simulink model "CompleteDronePathSimulation2"  (R2022b)
settings: Solver=VariableStepAuto  StartTime=0.0  StopTime=10.0  RelTol=1e-3
settings Model: Creator=zs  LastModifiedBy=zs

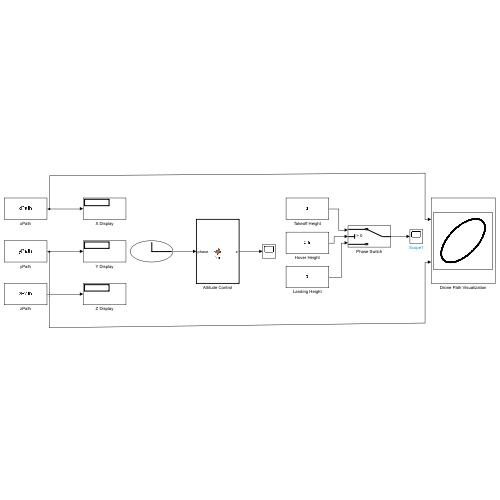
[thumbnail: Simulink's stored preview of the top-level diagram]
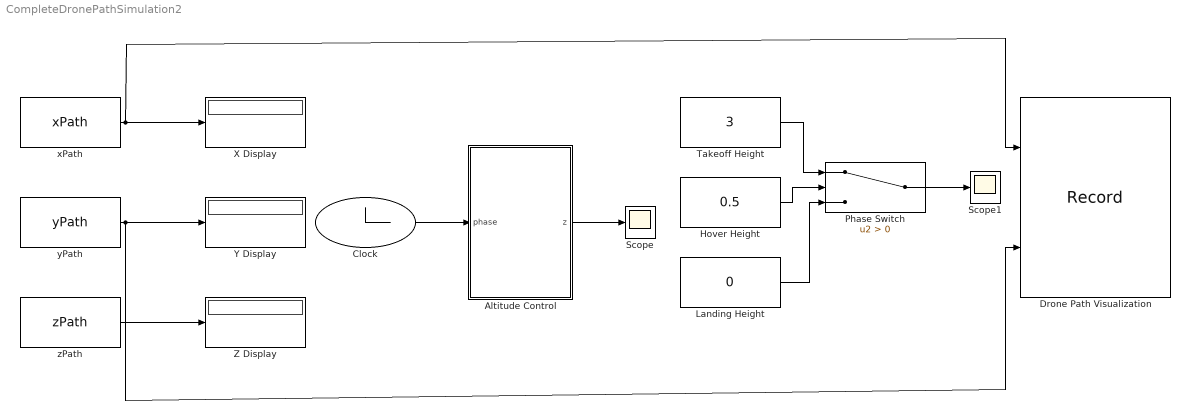
== system CompleteDronePathSimulation2 ==
  Altitude Control : MATLAB Function  TreatAsAtomicUnit=on
  Clock : Clock
  Drone Path Visualization : Record  FileSettingsInternal="{\"entries\":[{\"content\":{\"excelSettings\":{\"content\":{},\"type\":\"Streamout.ExcelSettings\"}},\"type\":\"Streamout.FileSettingStorage\",\"uuid\":\"701c7f2f-fa6d-4916-bfb4-89bd70d8efd9\"}],\"packageUris\":[\"http://schema.mathworks.com/mf0/streamout_blocks/R2020a\"],\"version\":\"1.0\"}"  Layout=[1 1]  SignalsInternal="{\"entries\":[{\"content\":{\"signals\":[{\"content\":{\"blockPath\":[\"CompleteDronePathSimulation2/Drone Path Visualization\"],\"channel\":[],\"dimensions\":[179],\"domain\":\"CompleteDronePathSimulation2/Drone Path Visualization\",\"hasChildren\":true,\"lineColor\":\"#edb120\",\"plots\":[],\"port\":1,\"sid\":[],\"signalID\":225,\"signalName\":\"xPath\"},\"type\":\"RecordBlkView.Signal\",\"uuid\":\"a3cad74d-0c4d-46ad-b448-e85591da0594\"},{\"content\":{\"blockPath\":[\"CompleteDronePathSimulation2/Drone Path Visualization\"],\"channel\":[1],\"dimensions\":[179],\"domain\":\"CompleteDronePathSimulation2/Drone Path Visualization\",\"lineColor\":\"#7e2f8e\",\"parentID\":225,\"plots\":[],\"port\":1,\"sid\":[],\"signalID\":226,\"signalName\":\"xPath\"},\"type\":\"RecordBlkView.Signal\",\"uuid\":\"7178f454-a0ae-4261-bb45-d0e300f4410c\"},{\"content\":{\"blockPath\":[\"CompleteDronePathSimulation2/Drone Path Visualization\"],\"channel\":[],\"dimensions\":[179],\"domain\":\"CompleteDronePathSimulation2/Drone Path Visualization\",\"hasChildren\":true,\"lineColor\":\"#77ac30\",\"plots\":[],\"port\":2,\"sid\":[],\"signalID\":408,\"signalName\":\"yPath\"},\"type\":\"RecordBlkView.Signal\",\"uuid\":\"60e1e068-7377-4912-8406-220e7cc34102\"},{\"content\":{\"blockPath\":[\"CompleteDronePathSimulation2/Drone Path Visualization\"],\"channel\":[1],\"dimensions\":[179],\"domain\":\"CompleteDronePathSimulation2/Drone Path Visualization\",\"lineColor\":\"#4dbeee\",\"parentID\":408,\"plots\":[],\"port\":2,\"sid\":[],\"signalID\":409,\"signalName\":\"yPath\"},\"type\":\"RecordBlkView.Signal\",\"uuid\":\"6962e288-c15f-4001-a316-d17ff70b3f4c\"}]},\"type\":\"RecordBlkView.InputSignals\",\"uuid\":\"a07fd186-7fd0-4c18-bff8-9bf155d2cde3\"}],\"packageUris\":[\"http://schema.mathworks.com/mf0/streamout_blocks/R2020a\"],\"version\":\"1.0\"}"  VisualizationBindings="{\"xyplotplugin\":{\"info\":[{\"series\":[],\"subplotID\":1}]}}"  CompatibilityTag=XY
  Hover Height : Constant  Value=0.5
  Landing Height : Constant  Value=0
  Phase Switch : Switch  Criteria=u2 > Threshold  SaturateOnIntegerOverflow=off  InputSameDT=off
  Scope : Scope
  Scope1 : Scope
  Takeoff Height : Constant  Value=3
  X Display : Display
  Y Display : Display
  Z Display : Display
  xPath : FromWorkspace  VariableName=xPath
  yPath : FromWorkspace  VariableName=yPath
  zPath : FromWorkspace  VariableName=zPath
  wires:
  xPath/1 -> X Display/1, Drone Path Visualization/1
  yPath/1 -> Y Display/1, Drone Path Visualization/2
  zPath/1 -> Z Display/1
  Clock/1 -> Altitude Control/1(phase)
  Takeoff Height/1 -> Phase Switch/1
  Hover Height/1 -> Phase Switch/2
  Landing Height/1 -> Phase Switch/3
  Phase Switch/1 -> Scope1/1
  Altitude Control/1(z) -> Scope/1

== matlab function CompleteDronePathSimulation2/Altitude Control ==
  data: phase input; z output
function z = fcn(phase)
    if phase == 1
        z = 3;       % Takeoff height
    elseif phase == 2
        z = 1.5;     % Hover height
    else
        z = 0;       % Landing height
    end
end
